simulink model "simulation_hw3"  (R2023b)
settings: Solver=ode4  StartTime=0.0  StopTime=60  FixedStep=0.001  RelTol=1e-3
settings Model: Creator=Dhiya  LastModifiedBy=Dhiya

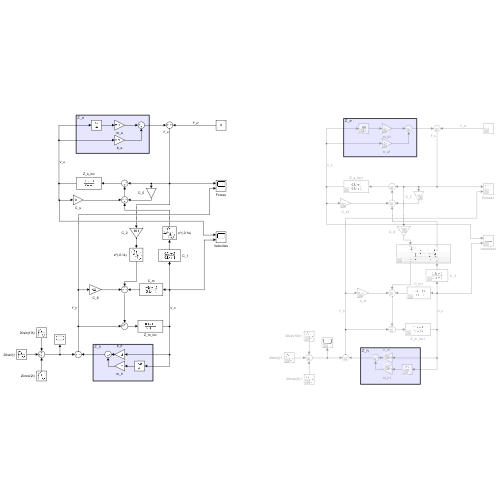
[thumbnail: Simulink's stored preview of the top-level diagram]
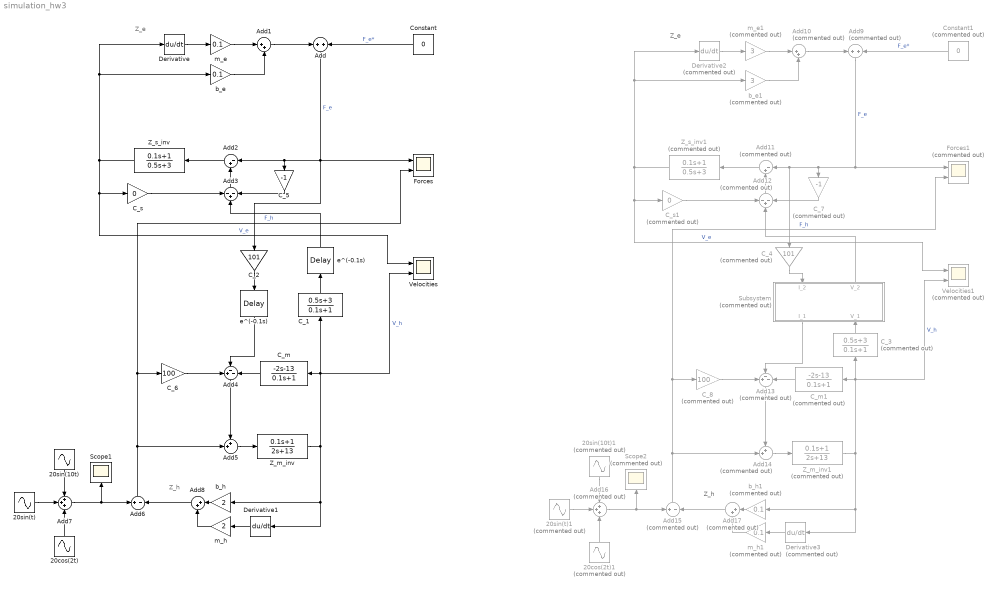
== system simulation_hw3 ==
  note: Z_h
  note: Z_e
  note: Z_h
  note: Z_e
  20cos(2t) : Sin  Amplitude=20  Frequency=2  Phase=pi/2  SampleTime=0
  20cos(2t)1 : Sin  Commented=on  Amplitude=20  Frequency=2  Phase=pi/2  SampleTime=0
  20sin(10t) : Sin  Amplitude=20  Frequency=10  SampleTime=0
  20sin(10t)1 : Sin  Commented=on  Amplitude=20  Frequency=10  SampleTime=0
  20sin(t) : Sin  Amplitude=20  SampleTime=0
  20sin(t)1 : Sin  Commented=on  Amplitude=20  SampleTime=0
  Add : Sum  Inputs=+|+
  Add1 : Sum  Inputs=|++
  Add10 : Sum  Commented=on  Inputs=|++
  Add11 : Sum  Commented=on  Inputs=|-+
  Add12 : Sum  Commented=on  Inputs=-+-
  Add13 : Sum  Commented=on  Inputs=+--
  Add14 : Sum  Commented=on  Inputs=++|
  Add15 : Sum  Commented=on  Inputs=+|-
  Add16 : Sum  Commented=on  Inputs=+++
  Add17 : Sum  Commented=on  Inputs=|++
  Add2 : Sum  Inputs=|-+
  Add3 : Sum  Inputs=-+-
  Add4 : Sum  Inputs=+--
  Add5 : Sum  Inputs=++|
  Add6 : Sum  Inputs=+|-
  Add7 : Sum  Inputs=+++
  Add8 : Sum  Inputs=|++
  Add9 : Sum  Commented=on  Inputs=+|+
  C_1 : TransferFcn  Numerator=[0.5 3]  Denominator=[0.1 1]
  C_2 : Gain  Gain=101
  C_3 : TransferFcn  Commented=on  Numerator=[0.5 3]  Denominator=[0.1 1]
  C_4 : Gain  Commented=on  Gain=101
  C_5 : Gain  Gain=-1
  C_6 : Gain  Gain=100
  C_7 : Gain  Commented=on  Gain=-1
  C_8 : Gain  Commented=on  Gain=100
  C_m : TransferFcn  Numerator=[-2 -13]  Denominator=[0.1 1]
  C_m1 : TransferFcn  Commented=on  Numerator=[-2 -13]  Denominator=[0.1 1]
  C_s : Gain  Gain=0
  C_s1 : Gain  Commented=on  Gain=0
  Constant : Constant  Value=0
  Constant1 : Constant  Commented=on  Value=0
  Derivative : Derivative
  Derivative1 : Derivative
  Derivative2 : Derivative  Commented=on
  Derivative3 : Derivative  Commented=on
  Forces : Scope  NumInputPorts=2
  Forces1 : Scope  Commented=on  NumInputPorts=2
  Scope1 : Scope
  Scope2 : Scope  Commented=on
  Subsystem : Subsystem  Commented=on
      settings: PortSchema="{\"entries\":[{\"content\":{\"sides\":[{\"content\":{\"connectorIds\":[\"In1\",\"Out2\"]},\"type\":\"ConnectorPlacement.EquallySpacedRectSide\",\"uuid\":\"b47614d8-4282-40b8-98b5-b63f244bcd96\"},{\"content\":{\"connectorIds\":[\"Out1\",\"In2\"],\"side\":\"RIGHT\"},\"type\":\"ConnectorPlacement.EquallySpacedRectSide\",\"uuid\":\"bd48739f-0f37-4abb-b4a6-b3e75c0b7ee5\"},{\"content\":{\"side\":\"TOP\"},\"type\":\"ConnectorPlacement.EquallySpacedRectSide\",\"uuid\":\"b94baccd-0b63-48fd-a532-2b1ed6a2ffaa\"}]},\"type\":\"ConnectorPlacement.EquallySpacedConnector\",\"uuid\":\"3afc87c5-143e-47c9-ba54-3d5bde851d7b\"}],\"packageUris\":[\"http://schema.mathworks.com/mf0/Connector/R2020b\"],\"version\":\"1.0\"}"
  Velocities : Scope  NumInputPorts=2
  Velocities1 : Scope  Commented=on  NumInputPorts=2
  Z_m_inv : TransferFcn  Numerator=[0.1 1]  Denominator=[2 13]
  Z_m_inv1 : TransferFcn  Commented=on  Numerator=[0.1 1]  Denominator=[2 13]
  Z_s_inv : TransferFcn  Numerator=[0.1 1]  Denominator=[0.5 3]
  Z_s_inv1 : TransferFcn  Commented=on  Numerator=[0.1 1]  Denominator=[0.5 3]
  b_e : Gain  Gain=0.1
  b_e1 : Gain  Commented=on  Gain=3
  b_h : Gain  Gain=2
  b_h1 : Gain  Commented=on  Gain=0.1
  e^(-0.1s) : TransportDelay  DelayTime=0.1
  "e^(-0.1s) " : TransportDelay  DelayTime=0.1
  m_e : Gain  Gain=0.1
  m_e1 : Gain  Commented=on  Gain=3
  m_h : Gain  Gain=2
  m_h1 : Gain  Commented=on  Gain=0.1
  wires:
  m_e/1 -> Add1/1
  b_e/1 -> Add1/2
  Derivative/1 -> m_e/1
  Z_s_inv/1 -> Velocities/1, C_s/1, Derivative/1, b_e/1  "V_e"
  Add/1 -> Forces/1, C_2/1, Add2/1, C_5/1  "F_e"
  Add2/1 -> Z_s_inv/1
  C_s/1 -> Add3/1
  C_5/1 -> Add3/3
  Add3/1 -> Add2/2
  C_1/1 -> e^(-0.1s)/1
  e^(-0.1s)/1 -> Add3/2
  C_2/1 -> "e^(-0.1s) "/1
  C_m/1 -> Add4/3
  Z_m_inv/1 -> b_h/1, Derivative1/1, Velocities/2, C_m/1, C_1/1  "V_h"
  Add4/1 -> Add5/1
  Add5/1 -> Z_m_inv/1
  C_6/1 -> Add4/1
  Add6/1 -> Add5/2, Forces/2, C_6/1  "F_h"
  Add7/1 -> Scope1/1, Add6/1
  20cos(2t)/1 -> Add7/3
  20sin(t)/1 -> Add7/2
  20sin(10t)/1 -> Add7/1
  Derivative1/1 -> m_h/1
  b_h/1 -> Add8/1
  m_h/1 -> Add8/2
  Constant/1 -> Add/2  "F_e*"
  "e^(-0.1s) "/1 -> Add4/2
  Add1/1 -> Add/1
  Add8/1 -> Add6/2
  Subsystem/1(I_1) -> Add13/2
  Subsystem/2(V_2) -> Add12/2
  Add17/1 -> Add15/2
  Add11/1 -> Z_s_inv1/1
  Constant1/1 -> Add9/2  "F_e*"
  Add10/1 -> Add9/1
  20cos(2t)1/1 -> Add16/3
  b_h1/1 -> Add17/1
  Add15/1 -> Add14/2, Forces1/2, C_8/1  "F_h"
  Derivative3/1 -> m_h1/1
  Add12/1 -> Add11/2
  20sin(10t)1/1 -> Add16/1
  20sin(t)1/1 -> Add16/2
  Add13/1 -> Add14/1
  m_h1/1 -> Add17/2
  Derivative2/1 -> m_e1/1
  Z_m_inv1/1 -> b_h1/1, Derivative3/1, Velocities1/2, C_m1/1, C_3/1  "V_h"
  C_m1/1 -> Add13/3
  Add16/1 -> Scope2/1, Add15/1
  C_8/1 -> Add13/1
  C_7/1 -> Add12/3
  C_s1/1 -> Add12/1
  Z_s_inv1/1 -> Velocities1/1, C_s1/1, Derivative2/1, b_e1/1  "V_e"
  m_e1/1 -> Add10/1
  Add14/1 -> Z_m_inv1/1
  Add9/1 -> C_4/1, Add11/1, C_7/1, Forces1/1  "F_e"
  C_3/1 -> Subsystem/2(V_1)
  C_4/1 -> Subsystem/1(I_2)
  b_e1/1 -> Add10/2

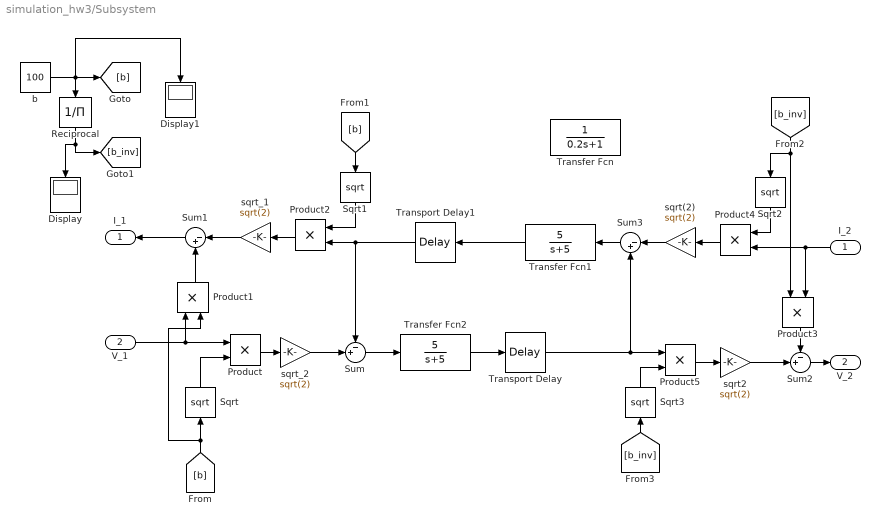
== system simulation_hw3/Subsystem ==
  I_2 : Inport
  V_1 : Inport  Port=2
  Display : Display
  Display1 : Display
      settings: Decimation=100
  Product{,1..5} (6 alike) : Product
  Reciprocal : Product  Inputs=/
  Sqrt{,1..3} (4 alike) : Sqrt
  Sum : Sum  Inputs=-+|
  Sum1 : Sum  Inputs=|-+
  Sum2 : Sum  Inputs=-+|
  Sum3 : Sum  Inputs=|-+
  Transfer Fcn : TransferFcn  Denominator=[0.2 1]
  Transfer Fcn1 : TransferFcn  Numerator=[5]  Denominator=[1 5]
  Transfer Fcn2 : TransferFcn  Numerator=[5]  Denominator=[1 5]
  Transport Delay : TransportDelay  DelayTime=0.1
  Transport Delay1 : TransportDelay  DelayTime=0.1
  b : Constant  Value=100
  sqrt(2) : Gain  Gain=sqrt(2)
  sqrt2 : Gain  Gain=sqrt(2)
  sqrt_1 : Gain  Gain=sqrt(2)
  sqrt_2 : Gain  Gain=sqrt(2)
  I_1 : Outport
  V_2 : Outport  Port=2
  wires:
  V_1/1 -> Product1/1, Product/1
  Product/1 -> sqrt_2/1
  sqrt_2/1 -> Sum/2
  Sqrt/1 -> Product/2
  Product1/1 -> Sum1/2
  sqrt_1/1 -> Sum1/1
  Product2/1 -> sqrt_1/1
  Transport Delay1/1 -> Sum/1, Product2/2
  b/1 -> Display1/1, [b], Reciprocal/1
  [b] -> Product1/2, Sqrt/1
  [b] -> Sqrt1/1
  Sqrt1/1 -> Product2/1
  Sum1/1 -> I_1/1
  Reciprocal/1 -> Display/1, [b_inv]
  I_2/1 -> Product3/2, Product4/2
  [b_inv] -> Sqrt2/1, Product3/1
  Product3/1 -> Sum2/1
  Sum2/1 -> V_2/1
  Sqrt2/1 -> Product4/1
  Product4/1 -> sqrt(2)/1
  sqrt(2)/1 -> Sum3/1
  Transport Delay/1 -> Product5/1, Sum3/2
  Product5/1 -> sqrt2/1
  [b_inv] -> Sqrt3/1
  Sqrt3/1 -> Product5/2
  sqrt2/1 -> Sum2/2
  Sum3/1 -> Transfer Fcn1/1
  Transfer Fcn1/1 -> Transport Delay1/1
  Sum/1 -> Transfer Fcn2/1
  Transfer Fcn2/1 -> Transport Delay/1
